simulink model "DIGITAL_CIRCUIT"  (R2025b)
settings: Solver=VariableStepAuto  StartTime=0.0  StopTime=1  RelTol=1e-3
settings Model: Creator=kalas  LastModifiedBy=kalas

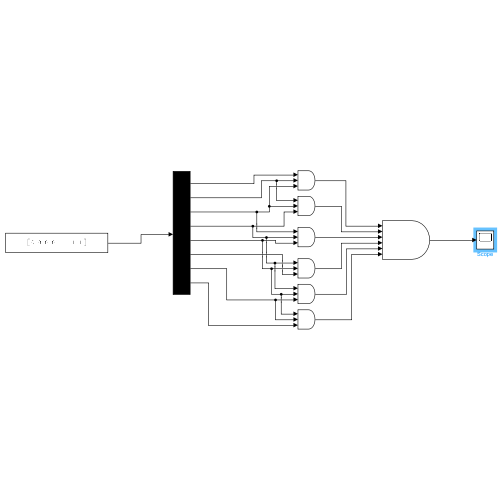
[thumbnail: Simulink's stored preview of the top-level diagram]
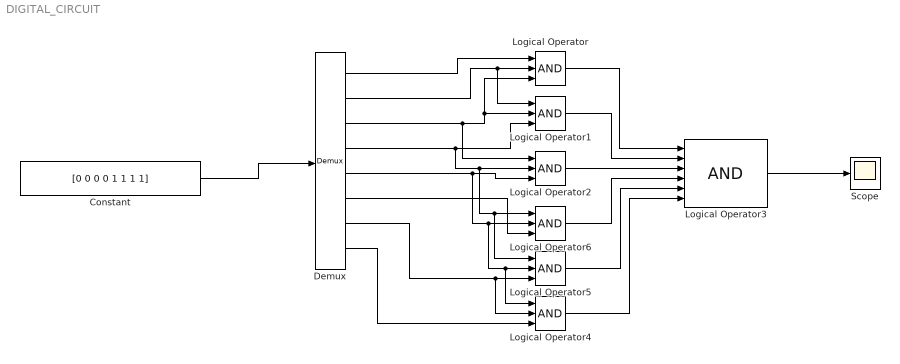
== system DIGITAL_CIRCUIT ==
  Constant : Constant  Value=[0 0 0 0 1 1 1 1]
  Demux : Demux  Outputs=8
  Logical Operator{,1..2,4..6} (6 alike) : Logic  Inputs=3  IconShape=distinctive  AllPortsSameDT=off  OutDataTypeStr=boolean
  Logical Operator3 : Logic  Inputs=6  IconShape=distinctive  AllPortsSameDT=off  OutDataTypeStr=boolean
  Scope : Scope
      settings: ActiveDisplayYMinimum=-1  ActiveDisplayYMaximum=1
  wires:
  Constant/1 -> Demux/1
  Demux/1 -> Logical Operator/1
  Demux/2 -> Logical Operator1/1, Logical Operator/2
  Demux/3 -> Logical Operator2/1, Logical Operator/3, Logical Operator1/2
  Demux/4 -> Logical Operator5/1, Logical Operator6/1, Logical Operator2/2, Logical Operator1/3
  Demux/6 -> Logical Operator6/3
  Demux/7 -> Logical Operator4/2, Logical Operator5/3
  Demux/8 -> Logical Operator4/3
  Demux/5 -> Logical Operator4/1, Logical Operator5/2, Logical Operator6/2, Logical Operator2/3
  Logical Operator/1 -> Logical Operator3/1
  Logical Operator1/1 -> Logical Operator3/2
  Logical Operator2/1 -> Logical Operator3/3
  Logical Operator6/1 -> Logical Operator3/4
  Logical Operator5/1 -> Logical Operator3/5
  Logical Operator4/1 -> Logical Operator3/6
  Logical Operator3/1 -> Scope/1
